simulink model "Project3_Q2"  (R2018a)
settings: Solver=FixedStepAuto  StartTime=0.0  StopTime=2  RelTol=1e-3
libraries: powerlib x12, powerlib_meascontrol x3, pePowerMeasurement x2
settings Model: Creator=ROG  LastModifiedBy=user

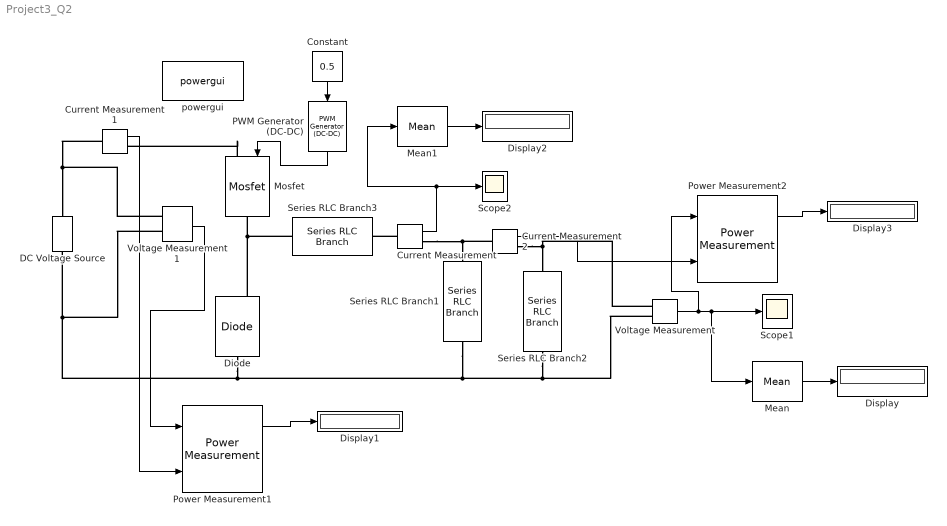
== system Project3_Q2 ==
  Constant : Constant  Value=0.5
  Current Measurement : powerlib/Measurements/Current Measurement  PhasorSimulation=off  OutputType=Complex  PSBequivalent=0
  Current Measurement1 : powerlib/Measurements/Current Measurement  PhasorSimulation=off  OutputType=Complex  PSBequivalent=0
  Current Measurement2 : powerlib/Measurements/Current Measurement  PhasorSimulation=off  OutputType=Complex  PSBequivalent=0
  DC Voltage Source : powerlib/Electrical Sources/DC Voltage Source  Amplitude=56  Measurements=None
  Diode : powerlib/Power Electronics/Diode  Ron=0.001  Lon=0  Vf=0.8  IC=0  UseSnubber=0  Rs=500  Cs=250e-9  Measurements=on
  Display{,1..3} (4 alike) : Display
  Mean : powerlib_meascontrol/Measurements/Mean  Freq=50  Vinit=0  Ts=0
  Mean1 : powerlib_meascontrol/Measurements/Mean  Freq=50  Vinit=0  Ts=0
  Mosfet : powerlib/Power Electronics/Mosfet  Ron=0.02  Lon=0  Rd=0.01  Vfd=0.74  IC=0  Rs=1e5  Cs=inf  Measurements=off
  PWM Generator (DC-DC) : powerlib_meascontrol/Pulse & Signal Generators/PWM Generator (DC-DC)  Fsw=20000  Ts=0
  Power Measurement1 : pePowerMeasurement/Power Measurement  OverrideUsingVariant=Continuous  F=60  K=[0 1 2 3]  Ts=0
  Power Measurement2 : pePowerMeasurement/Power Measurement  OverrideUsingVariant=Continuous  F=60  K=[0 1 2 3]  Ts=0
  Scope1 : Scope
  Scope2 : Scope
  Series RLC Branch1 : powerlib/Elements/Series RLC Branch  LConnTagsString=__new0  RConnTagsString=__new0  BranchType=RC  Resistance=67e-3  Inductance=1e-3  SetiL0=off  InitialCurrent=0  Capacitance=75e-5  Setx0=off  InitialVoltage=0  Measurements=None
  Series RLC Branch2 : powerlib/Elements/Series RLC Branch  LConnTagsString=__new0  RConnTagsString=__new0  BranchType=R  Resistance=4  Inductance=1e-3  SetiL0=off  InitialCurrent=0  Capacitance=1e-6  Setx0=off  InitialVoltage=0  Measurements=None
  Series RLC Branch3 : powerlib/Elements/Series RLC Branch  LConnTagsString=__new0  RConnTagsString=__new0  BranchType=RL  Resistance=49e-3  Inductance=33e-5  SetiL0=off  InitialCurrent=0  Capacitance=1e-6  Setx0=off  InitialVoltage=0  Measurements=None
  Voltage Measurement : powerlib/Measurements/Voltage Measurement  PhasorSimulation=off  OutputType=Complex  PSBequivalent=0
  Voltage Measurement1 : powerlib/Measurements/Voltage Measurement  PhasorSimulation=off  OutputType=Complex  PSBequivalent=0
  powergui : powerlib/powergui  Priority=1  SimulationMode=Discrete  SampleTime=1e-6  frequency=60  Iterations=50  frequencyindice=0  Pbase=100e6  ErrMax=1e-4  UnitsV=kV  UnitsW=MW  buscounter=0  FunctionMessages=off  echomessages=off  EnableUseOfTLC=off  CurrentSourceSwitches=off  DisableSnubberDevices=off  DisableRonSwitches=off  DisableVfSwitches=off  DisplayEquations=off  SolverType=Tustin/Backward Euler (TBE)  Interpol=off  ExternalGateDelay=off  methode=off  Ts=100  x0status=blocks  SPID=off  SwTol=0  HookPort=off  RestoreLinks=warning  ResistiveCurrentMeasurement=off  Frange=[0:2:500]  Ylog=off  Xlog=on  ShowGrid=off  save=off  variable=ZData  structure=0  ZoomFFT=off  StartTime=0.0  cycles=1  DisplayStyle=1  fundamental=60  FreqAxis=off  MaxFrequency=1000  frequencyindicesteady=1  RmsSteady=1  display=off
  wires:
  Constant/1 -> PWM Generator (DC-DC)/1
  PWM Generator (DC-DC)/1 -> Mosfet/1
  Mean/1 -> Display/1
  Current Measurement/1 -> Mean1/1, Scope2/1
  Mean1/1 -> Display2/1
  Current Measurement2/1 -> Power Measurement2/2
  Voltage Measurement/1 -> Power Measurement2/1, Mean/1, Scope1/1
  Power Measurement2/1 -> Display3/1
  Voltage Measurement1/1 -> Power Measurement1/1
  Current Measurement1/1 -> Power Measurement1/2
  Power Measurement1/1 -> Display1/1
  connections:
  Series RLC Branch2/RConn1 -- Voltage Measurement/LConn2 -- Series RLC Branch1/RConn1 -- Voltage Measurement1/LConn2 -- DC Voltage Source/LConn1 -- Diode/LConn1
  Current Measurement/RConn1 -- Current Measurement2/LConn1 -- Series RLC Branch1/LConn1
  Series RLC Branch3/RConn1 -- Diode/RConn1 -- Mosfet/RConn1
  Current Measurement/LConn1 -- Series RLC Branch3/LConn1
  Mosfet/LConn1 -- Current Measurement1/RConn1
  Current Measurement1/LConn1 -- Voltage Measurement1/LConn1 -- DC Voltage Source/RConn1
  Voltage Measurement/LConn1 -- Current Measurement2/RConn1 -- Series RLC Branch2/LConn1
